simulink model "Project1"  (R2021a)
settings: Solver=VariableStepAuto  StartTime=0.0  StopTime=10.0  MaxStep=0.01  RelTol=1e-3
settings Model: Creator=se7en  LastModifiedBy=se7en

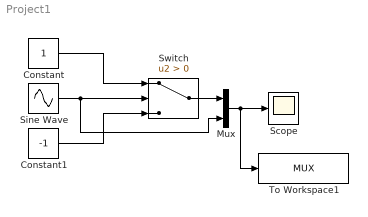
== system Project1 ==
  Constant : Constant
  Constant1 : Constant  Value=-1
  Mux : Mux  Inputs=2
  Scope : Scope
  Sine Wave : Sin  SampleTime=0
  Switch : Switch  Criteria=u2 > Threshold
  To Workspace1 : ToWorkspace  VariableName=MUX  SaveFormat=Timeseries  SampleTime=-1
  wires:
  Sine Wave/1 -> Mux/2, Switch/2
  Constant/1 -> Switch/1
  Constant1/1 -> Switch/3
  Switch/1 -> Mux/1
  Mux/1 -> To Workspace1/1, Scope/1
